simulink model "Sensors"  (R2020a)
settings: Solver=VariableStepAuto  StartTime=0.0  StopTime=10.0  RelTol=1e-3
settings Model: Creator=Administrator  LastModifiedBy=Administrator

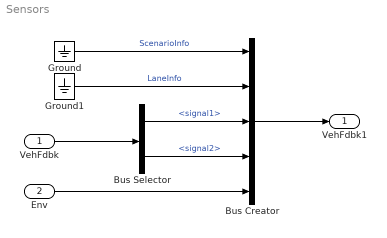
== system Sensors ==
  VehFdbk : Inport
  Env : Inport  Port=2
  Bus Creator : BusCreator  Inputs=5
  Bus Selector : BusSelector  OutputSignals=signal1,signal2
  Ground : Ground
  Ground1 : Ground
  VehFdbk1 : Outport
  wires:
  Ground/1 -> Bus Creator/1  "ScenarioInfo"
  Ground1/1 -> Bus Creator/2  "LaneInfo"
  VehFdbk/1 -> Bus Selector/1
  Env/1 -> Bus Creator/5
  Bus Creator/1 -> VehFdbk1/1
  Bus Selector/1 -> Bus Creator/3  "<signal1>"
  Bus Selector/2 -> Bus Creator/4  "<signal2>"
